simulink model "servo_system_complete"  (R2021a)
settings: Solver=FixedStepAuto  StartTime=0.0  StopTime=t_end  FixedStep=T_s  RelTol=1e-3
undefined symbols (not defined in the file): Amp, angle_ini, b1, b2, displacement, home, K, K_sensor, Kb1, Kb2, Kd1, Kd2, Ki1, Ki2, Kp1, Kp2, L1, L2, m1, m2, mL, mM2, mode, phi, Ra1, Ra2, sampling, T, T_s, X, Y, Z
libraries: sm_lib x56, fl_lib x28, nesl_utility x27, ee_lib x7, simulink x2, pid_lib x2
(part 3 of 3)

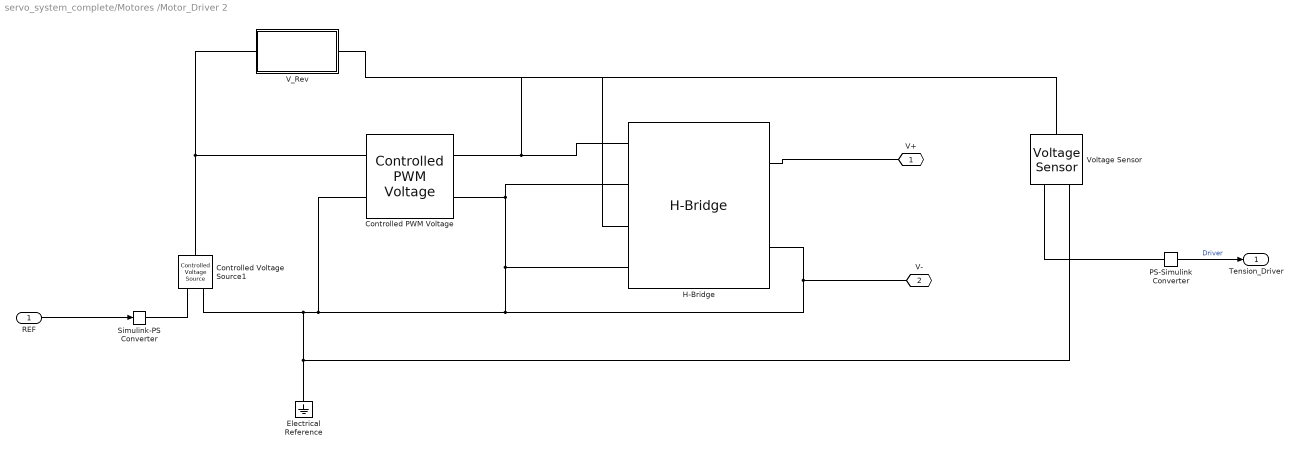
== system servo_system_complete/Motores /Motor_Driver 2 ==
  REF : Inport
  Controlled PWM Voltage : ee_lib/Integrated Circuits/Controlled PWM Voltage  F=4000 Hz  TD=0 s  pulse_width_offset=0 s  pulse_min=0 s  Vmin=0 V  Vmax=10 V  Vm=12 V  pwm_or_av=1  event_type=1  sample_time=1e-6 s  u_min=0  u_max=1
  Controlled Voltage Source1 : fl_lib/Electrical/Electrical Sources/Controlled Voltage Source
  Electrical Reference : fl_lib/Electrical/Electrical Elements/Electrical Reference
  H-Bridge : ee_lib/Semiconductors & Converters/Converters/H-Bridge  supply_ports=ee.enum.supply_ports.hidesupply  Venable=2.5 V  Vmax=12 V  Vreverse=2.5 V  Vbrake=2.5 V  Vm=12 V  pwm_or_av=ee.enum.pwm_or_av.pwm  regenerative_braking_mode=ee.enum.converters.regenerative_braking_mode.always_enabled  discontinuous=ee.enum.current_profile.continuous  freewheeling_mode=ee.enum.converters.freewheeling_mode.one_switch_one_diode  Ron=0.1 Ohm  Don=0.05 Ohm  Goff=1e-6 S  Rload=10 Ohm  Lload=1e-5 H  F=10 kHz  thermal_mass=100 J/K  initial_temperature=298.15 K  Ron2=0.1 Ohm  Don2=0.05 Ohm  Tmeas=298.15 K  Tmeas2=398.15 K
  PS-Simulink Converter : nesl_utility/PS-Simulink Converter  PhysicalDomain=network_engine_domain  SubClassName=ps_output  LeftPortType=input  RightPortType=output  PseudoPeriodic=off  Frequencies=[]  Unit=V  AffineConversion=off
      settings: SourceProductBaseCode=PW,SS
  Simulink-PS Converter : nesl_utility/Simulink-PS Converter  PhysicalDomain=network_engine_domain  SubClassName=ps_input  LeftPortType=input  RightPortType=output  PseudoPeriodic=off  Frequencies=[]  NoiseDistribution=none  NoiseParameters=[]  Unit=V  AffineConversion=off  FilteringAndDerivatives=provide  SimscapeFilterOrder=1  InputFilterTimeConstant=0.001  UdotUserProvided=0
      settings: SourceProductBaseCode=PW,SS
  V_Rev : Subsystem
  Voltage Sensor : fl_lib/Electrical/Electrical Sensors/Voltage Sensor
  V+ : PMIOPort  Side=Right
  V- : PMIOPort  Port=2  Side=Right
  Tension_Driver : Outport
  wires:
  REF/1 -> Simulink-PS Converter/1
  PS-Simulink Converter/1 -> Tension_Driver/1  "Driver"
  connections:
  V+/RConn1 -- H-Bridge/RConn1
  V_Rev/LConn1 -- Controlled PWM Voltage/LConn1 -- Controlled Voltage Source1/LConn1
  H-Bridge/RConn2 -- V-/RConn1 -- Controlled PWM Voltage/LConn2 -- Voltage Sensor/RConn2 -- Electrical Reference/LConn1 -- Controlled Voltage Source1/RConn2 -- H-Bridge/LConn2 -- Controlled PWM Voltage/RConn2 -- H-Bridge/LConn4
  Simulink-PS Converter/RConn1 -- Controlled Voltage Source1/RConn1
  Controlled PWM Voltage/RConn1 -- H-Bridge/LConn1 -- Voltage Sensor/LConn1
  Voltage Sensor/RConn1 -- PS-Simulink Converter/LConn1
  V_Rev/RConn1 -- H-Bridge/LConn3

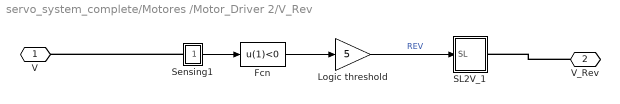
== system servo_system_complete/Motores /Motor_Driver 2/V_Rev ==
  Fcn : Fcn  Expr=u(1)<0
  Logic threshold : Gain  Gain=5
  SL2V_1 : Subsystem
  Sensing1 : Subsystem
      mask Display: disp('V')
  V : PMIOPort  Side=Left
  V_Rev : PMIOPort  Port=2  Side=Right
  wires:
  Logic threshold/1 -> SL2V_1/1(SL)  "REV"
  Fcn/1 -> Logic threshold/1
  Sensing1/1(Out1) -> Fcn/1
  connections:
  Sensing1/LConn1 -- V/RConn1
  V_Rev/RConn1 -- SL2V_1/RConn1

== system servo_system_complete/Motores /Motor_Driver 2/V_Rev/SL2V_1 ==
  SL : Inport
  Controlled Voltage Source : fl_lib/Electrical/Electrical Sources/Controlled Voltage Source
  Electrical Reference : fl_lib/Electrical/Electrical Elements/Electrical Reference
  Simulink-PS Converter : nesl_utility/Simulink-PS Converter  PhysicalDomain=network_engine_domain  SubClassName=ps_input  LeftPortType=input  RightPortType=output  PseudoPeriodic=off  Frequencies=[]  NoiseDistribution=none  NoiseParameters=[]  Unit=V  AffineConversion=off  FilteringAndDerivatives=zero  SimscapeFilterOrder=1  InputFilterTimeConstant=.001  UdotUserProvided=0
      settings: SourceProductBaseCode=PW,SS
  V : PMIOPort  Side=Right
  wires:
  SL/1 -> Simulink-PS Converter/1
  connections:
  V/RConn1 -- Controlled Voltage Source/LConn1
  Simulink-PS Converter/RConn1 -- Controlled Voltage Source/RConn1
  Electrical Reference/LConn1 -- Controlled Voltage Source/RConn2

== system servo_system_complete/Motores /Motor_Driver 2/V_Rev/Sensing1 ==
  ERef13 : fl_lib/Electrical/Electrical Elements/Electrical Reference
  PS-Simulink Converter 2 : nesl_utility/PS-Simulink Converter  PhysicalDomain=network_engine_domain  SubClassName=ps_output  LeftPortType=input  RightPortType=output  PseudoPeriodic=off  Frequencies=[]  Unit=V  AffineConversion=off
      settings: SourceProductBaseCode=PW,SS
  Voltage Sensor : fl_lib/Electrical/Electrical Sensors/Voltage Sensor
  V : PMIOPort  Side=Left
  Out1 : Outport  VectorParamsAs1DForOutWhenUnconnected=off
  wires:
  PS-Simulink Converter 2/1 -> Out1/1
  connections:
  V/RConn1 -- Voltage Sensor/LConn1
  Voltage Sensor/RConn2 -- ERef13/LConn1
  Voltage Sensor/RConn1 -- PS-Simulink Converter 2/LConn1

== matlab function servo_system_complete/Subsystem/inverse_kinematic ==
  data: t input; T input; L1 input; L2 input; displacement input; home input; theta1 output; theta2 output; angle_ini input; Amp input; phi input; K input
function [theta1,theta2]=inverse_kinematic(t,T,L1,L2, displacement,home,angle_ini,Amp,phi,K) 

% Distancia [cm]
desp_x=displacement(1);
desp_y=displacement(2);

x_home=home(1); 
y_home=home(2);

r_base=7.5;       % radio base [cm]

r_max=Amp*r_base*(1+K);

% Tiempo Desplazamiento inicial
r_ini=Amp*r_base*(1-K*cos(4*angle_ini+phi));

[x,y]=pol2cart(angle_ini,r_ini);  

x=x+desp_x;   y=y+desp_y;

d=sqrt((x-x_home).^2+(y-y_home).^2);
vel=(r_base*2*pi/T);

t_start=d/vel;

angle=2*pi*(t-t_start)/T + angle_ini;

% Tiempo Desplazamiento inicial
r=Amp*r_base*(1-K*cos(4*angle+phi));

[x,y]=pol2cart(angle,r);  

x=x+desp_x;   y=y+desp_y;



if(t<t_start)  
  % Desplazamiento inicial
  sig2=1./(1+exp(-14*(t./t_start-0.5)));
  x=x_home+(x-x_home)*sig2;
  y=y_home+(y-y_home)*sig2;
end

[angle,r]=cart2pol(x,y);
L=sqrt(x.^2+y.^2);

% perfil de movimiento
theta=[angle-acos((L.^2+L1^2-L2^2)./(2*L*L1));
             acos((L.^2-L1^2-L2^2)/(2*L1*L2))];
theta1=theta(1);
theta2=theta(2);

end
